simulink model "pwm duty cycle"  (R2021a)
settings: Solver=VariableStepAuto  StartTime=0.0  StopTime=10.0  RelTol=1e-3
libraries: spsMeanLib x3
settings Model: Creator=hritw  LastModifiedBy=hritw

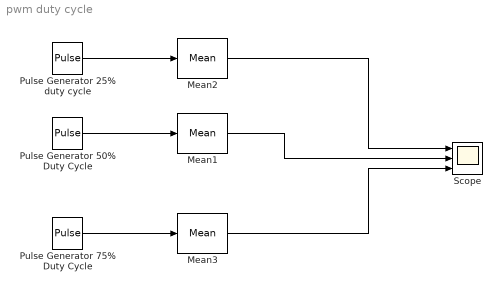
== system pwm duty cycle ==
  Mean1 : spsMeanLib/Mean  Freq=0.25  Vinit=0  Ts=0
  Mean2 : spsMeanLib/Mean  Freq=0.25  Vinit=0  Ts=0
  Mean3 : spsMeanLib/Mean  Freq=0.25  Vinit=0  Ts=0
  Pulse Generator 25% duty cycle : DiscretePulseGenerator  PulseType=Time based  Amplitude=4  Period=4  PulseWidth=25
  Pulse Generator 50% Duty Cycle : DiscretePulseGenerator  PulseType=Time based  Amplitude=4  Period=4  PulseWidth=50
  Pulse Generator 75% Duty Cycle : DiscretePulseGenerator  PulseType=Time based  Amplitude=4  Period=4  PulseWidth=75
  Scope : Scope  NumInputPorts=3
  wires:
  Pulse Generator 25% duty cycle/1 -> Mean2/1
  Pulse Generator 75% Duty Cycle/1 -> Mean3/1
  Pulse Generator 50% Duty Cycle/1 -> Mean1/1
  Mean3/1 -> Scope/3
  Mean2/1 -> Scope/1
  Mean1/1 -> Scope/2
